simulink model "generic_Truck_And_Trailer"  (R2025a)
settings: Solver=VariableStepAuto  StartTime=0.0  StopTime=350  FixedStep=0.01  MaxStep=0.001  RelTol=1e-3  EnableMultiTasking=on
libraries: TruckMaker4SL x250, simulink x1
(part 7 of 11)

== matlab function generic_Truck_And_Trailer/TruckMaker/Subsystem1/ONE_TRACK_MODEL_TRACTOR_UKF/UKF_ONE_TRACK_TruckAndTrailer ==
  data: z input; u input; xhat output; Q input; R input; Ts input; P output; dxdt output; innovation output; K_out output; S_out output; z_pred_out output; data input; truck_Ff output; truck_Fr output; trailer_v_hitch output; trailer_v_axle output; trailer_F_hitch output; trailer_F_tire output; truck_v_hitch output
function [xhat, P, dxdt, innovation, K_out, S_out, z_pred_out,truck_Ff,truck_Fr, trailer_v_hitch,trailer_v_axle,trailer_F_hitch,trailer_F_tire,truck_v_hitch] = UKF_TruckTrailer(z,u,Q,R,Ts,data)

persistent x Pk dxdt_old t
%% =========================
%% INIT
%% =========================
if isempty(x)
    x = [15;0.1;0.1;14;14;0;0;5]; % [vx vy wz Cf Cr psi wz_tr Cr_tr]
end
if isempty(Pk)
    Pk = diag([0.1 0.1 0.1 5 5 0.03 0.1 5]);
end
if isempty(dxdt_old)
    dxdt_old = zeros(8,1);
end
if isempty(t)
    t = 0;
end
t = data;
if t < 30
    xhat=x; P=Pk; dxdt=dxdt_old;
    
    innovation=zeros(length(z),1);
    K_out=zeros(length(x), length(z));
    S_out=eye(length(z));
    z_pred_out=zeros(length(z),1);
    
    trailer_v_axle   = zeros(3,1);
    trailer_v_hitch = zeros(3,1);
    truck_Ff = zeros(2,1);
    truck_Fr = zeros(2,1);
    truck_v_hitch=zeros(3,1);
    
    trailer_F_hitch = zeros(2,1);
    trailer_F_tire = zeros(2,1);
    
    return
end

%% =========================
%% CONSTANTS
%% =========================
g = 9.82;
% Truck
m = 6800; 
Jz = 12994.917; 
Rwheel = 0.50;
w_track = 2.1; 
% Trailer
m_tr = 31960;
Jz_tr = 145971.764;
% Geometry & koordinat punkter på Truck
p_cog = [3.473;0;0.925];
p_fax = [4.520;0;0.49];
p_rax = [0.950;0;0.49];
p_imu = [3.600;0;1.000];
hitch = [1.9;0;1.21];
Rcog = p_imu - p_cog;
hHitch= hitch(3);
lf = abs(p_fax(1)-p_cog(1)); 
lr = abs(p_cog(1)-p_rax(1)); 
L = lf + lr;
h = p_cog(3);
Rfax = p_fax - p_cog; Rfax(3)=-p_cog(3);
Rrax = p_rax - p_cog; Rrax(3)=-p_cog(3);
Rhitch = hitch - p_cog;
lhitch = Rhitch(1);
% Geometry Trailer
p_cog_tr = [-6.195;0;1.95];
p_rFax_tr = [-7.75;0;0.49];
p_rMax_tr = [-9.0;0;0.49];
p_rRax_tr = [-10.25;0;0.49];
hitch_tr = [-1.25;0;1.25];

% Avstånd från hitch till trailer-punkter
lf_h_tr = abs(hitch_tr(1)-p_cog_tr(1));
lr_f_tr = abs(p_cog_tr(1)-p_rFax_tr(1));
lr_m_tr = abs(p_cog_tr(1)-p_rMax_tr(1));
lr_r_tr = abs(p_cog_tr(1)-p_rRax_tr(1));
L_tr = lf_h_tr + lr_m_tr; % Hävarm till mittaxel

% Vektorer från trailer-CoG till axlar (för cross-product)
Frax_tr = p_rFax_tr - p_cog_tr; Frax_tr(3) = -p_cog_tr(3);
Mrax_tr = p_rMax_tr - p_cog_tr; Mrax_tr(3) = -p_cog_tr(3);
Rlrax_tr = p_rRax_tr - p_cog_tr; Rlrax_tr(3) =-p_cog_tr(3);
Rhitch_tr = hitch_tr - p_cog_tr; Rhitch_tr(3) = -abs(hitch_tr(3)-p_cog_tr(3));

h_cog_tr = p_cog_tr(3);

% Statisk load transfer parametrar (beräknas en gång)
l_1 = -lr_f_tr; l_2 = -lr_m_tr; l_3 = -lr_r_tr;
l_h = lf_h_tr;
mg_tr = m_tr * g;
denom = l_1 + l_2 + l_3 - 3*l_h;

%% =========================
%% INPUTS
%% =========================
delta = u(1); 
T_rl  = u(2);   
T_rr  = u(3);
Fxh   = u(4); 
Fx_f_brake  = -abs(u(6)) / Rwheel; 
Fx_r_brake  = -abs(u(7)) / Rwheel;
Fx_vehicle  = (T_rl+T_rr)/Rwheel + Fx_r_brake +Fx_f_brake;

%% =========================
%% UKF PARAMS
%% =========================
n = length(x);
nSPx = 2*n+1;
W0 = 1 - n/3;
Wi = (1 - W0)/(2*n);
gamma = sqrt(n/(1 - W0));

%% =========================
%% SIGMA POINTS (PRIOR)
%% =========================
Pk = (Pk+Pk')/2 + 1e-9*eye(n);
Sx = chol(Pk,'lower');
X_pre = zeros(n,nSPx);
X_pre(:,1) = x;
for i=1:n
    X_pre(:,i+1)   = x + gamma*Sx(:,i);
    X_pre(:,i+1+n) = x - gamma*Sx(:,i);
end

%% =========================
%% PREDICTION
%% =========================
X_pred = zeros(n,nSPx);
dxdt_model = zeros(n,1);
truck_Ff = zeros(2,1);
truck_Fr = zeros(2,1);
truck_v_hitch = zeros(3,1);
    
trailer_v_axle = zeros(3,1);
trailer_v_hitch = zeros(3,1);
trailer_F_hitch = zeros(2,1);
trailer_F_tire = zeros(2,1);

for k=1:nSPx
    Xk = X_pre(:,k);
    vx=Xk(1); vy=Xk(2); wz=Xk(3); Cf=Xk(4); Cr=Xk(5);
    psi=Xk(6); wz_tr=Xk(7); Cr_tr=Xk(8);
    
    v_cog=[vx;vy;0];
    omega=[0;0;wz];
    
    %% ===== TRAILER =====
    v_hitch_truck = v_cog + cross(omega,Rhitch);
    
    Rot_tr=[cos(psi) -sin(psi) 0;
            sin(psi) cos(psi)  0; 
              0         0      1];
   
    v_hitch_trailer = Rot_tr' * v_hitch_truck;
    
    % *** STATISK LOAD TRANSFER (Axels metod) ***
    Fz_hitch = (mg_tr * (l_1 + l_2 + l_3)) / denom;
    Fz_tr_each = -(l_h * mg_tr) / denom;
    
    % Begränsa till fysiska värden
    Fz_hitch = max(100, min(Fz_hitch, m_tr*g));
    Fz_tr_each = max(100, min(Fz_tr_each, m_tr*g));

    % Hastigheter och slip för traileraxlar (relativt trailer CoG)
    omega_tr = [0;0;wz_tr];
    v_cog_tr = v_hitch_trailer - cross(omega_tr, Rhitch_tr);
    
    v_tr_f = v_cog_tr + cross(omega_tr, Frax_tr);
    v_tr_m = v_cog_tr + cross(omega_tr, Mrax_tr);
    v_tr_r = v_cog_tr + cross(omega_tr, Rlrax_tr);  
    
    alpha_tr_f = atan2(v_tr_f(2), max(abs(v_tr_f(1)), 0.1));
    alpha_tr_m = atan2(v_tr_m(2), max(abs(v_tr_m(1)), 0.1));
    alpha_tr_r = atan2(v_tr_r(2), max(abs(v_tr_r(1)), 0.1));
    
    Fy_f_tr = -Cr_tr * alpha_tr_f * Fz_tr_each;
    Fy_m_tr = -Cr_tr * alpha_tr_m * Fz_tr_each;
    Fy_r_tr = -Cr_tr * alpha_tr_r * Fz_tr_each;
    
    % Hitch-kraft (momentjämvikt)
    Fyh_mod = (Fy_f_tr*lr_f_tr + Fy_m_tr*lr_m_tr + Fy_r_tr*lr_r_tr) / (L_tr);
     
    if k==1
        trailer_v_hitch = v_hitch_trailer;
        trailer_v_axle = v_tr_m;
        truck_v_hitch = v_hitch_truck;
        trailer_F_hitch = [Fyh_mod; Fz_hitch];
        trailer_F_tire = [Fy_m_tr; Fz_tr_each];
    end

    %% ===== TRUCK =====
    % Transformera hitch-krafter till Truckens system
    F_hitch_body = Rot_tr * [Fxh; Fyh_mod; 0];
    
    Rotf=[cos(delta) -sin(delta)  0; 
          sin(delta)  cos(delta)  0;
              0           0       1];
    vf = Rotf'*(v_cog + cross(omega,Rfax));
    vr = v_cog + cross(omega,Rrax);
    
    alpha_f = atan2(vf(2),max(abs(vf(1)),0.1));
    alpha_r = atan2(vr(2),max(abs(vr(1)),0.1));
    
    % Vertikallast Truck
    ax_est = (Fx_vehicle - F_hitch_body(1))/m; 
    Ffz = (m*g*lr - m*ax_est*h + Fz_hitch*(hitch(1) - p_rax(1)) - F_hitch_body(1)*hHitch) / L;
    Frz = (m*g*lf + m*ax_est*h + Fz_hitch*(p_fax(1) - hitch(1)) + F_hitch_body(1)*hHitch) / L;
    
    Fy_f = -Cf * alpha_f * Ffz;
    Fy_r = -Cr * alpha_r * Frz;
    
    %% ===== DYNAMICS =====
    dvx = (Fx_vehicle - Fy_f*sin(delta) - F_hitch_body(1))/m + vy*wz;
    dvy = (Fy_f*cos(delta) + Fy_r - F_hitch_body(2))/m - vx*wz;
    dwz = (lf*Fy_f*cos(delta) - lr*Fy_r - lhitch*F_hitch_body(2))/Jz;
    
    dpsi = wz_tr - wz;  % Rätt tecken!
    
    % Moment kring trailer Cog
    dwz_tr = (lf_h_tr*Fyh_mod - lr_f_tr*Fy_f_tr - lr_m_tr*Fy_m_tr - lr_r_tr*Fy_r_tr)/Jz_tr;
    
    if k==1
        dxdt_model=[dvx;dvy;dwz;0;0;dpsi;dwz_tr;0];
        truck_Ff = [Fy_f;Ffz];
        truck_Fr = [Fy_r;Frz];
    end
    X_pred(:,k) = Xk + Ts*[dvx; dvy; dwz; 0; 0; dpsi; dwz_tr; 0];
end

%% ===== MEAN & COV
x_pred=zeros(n,1);
for k=1:nSPx
    w=(k==1)*W0+(k>1)*Wi;
    x_pred=x_pred+w*X_pred(:,k);
end
P_pred=zeros(n);
for k=1:nSPx
    w=(k==1)*W0+(k>1)*Wi;
    dx=X_pred(:,k)-x_pred;
    P_pred=P_pred+w*(dx*dx');
end
P_pred=P_pred+Q*Ts;

%% =========================
%% MEASUREMENT UPDATE
%% =========================
Sx=chol((P_pred+P_pred')/2 + 1e-9*eye(n),'lower');
X_post=zeros(n,nSPx);
X_post(:,1)=x_pred;
for i=1:n
    X_post(:,i+1)  =x_pred + gamma*Sx(:,i);
    X_post(:,i+1+n)=x_pred - gamma*Sx(:,i);
end

Z=zeros(10,nSPx);
for k=1:nSPx
    Xk=X_post(:,k);
    vx=Xk(1); vy=Xk(2); wz=Xk(3); Cf=Xk(4); Cr=Xk(5);
    psi=Xk(6); wz_tr=Xk(7); Cr_tr=Xk(8); 

    v_cog=[vx;vy;0];
    omega=[0;0;wz];
    
    % *** SAMMA STATISKA LOAD TRANSFER som i prediction ***
    Fz_hitch_meas = (mg_tr * (l_1 + l_2 + l_3)) / denom;
    Fz_tr_each_meas = -(l_h * mg_tr) / denom;
    
    Fz_hitch_meas = max(100, min(Fz_hitch_meas, m_tr*g));
    Fz_tr_each_meas = max(100, min(Fz_tr_each_meas, m_tr*g));
    
    % Upprepa kraftberäkning för z_pred
    Rot_tr=[cos(psi) -sin(psi) 0;
            sin(psi)  cos(psi) 0;
                0       0      1];

    v_hitch_tr = Rot_tr' * ([vx;vy;0] + cross([0;0;wz],Rhitch));
    
    % Samma logik som i prediction
    v_cog_tr_meas = v_hitch_tr - cross([0;0;wz_tr], Rhitch_tr);
    v_tr_m_meas = v_cog_tr_meas + cross([0;0;wz_tr], Mrax_tr);
    alpha_tr_m = atan2(v_tr_m_meas(2), max(abs(v_tr_m_meas(1)), 0.1));
    Fy_m_tr_meas = -Cr_tr * alpha_tr_m * Fz_tr_each_meas;
   
    % Beräkna Fy_f_tr och Fy_r_tr för hitch-kraften
    v_tr_f_meas = v_cog_tr_meas + cross([0;0;wz_tr], Frax_tr);
    v_tr_r_meas = v_cog_tr_meas + cross([0;0;wz_tr], Rlrax_tr);
    alpha_tr_f_meas = atan2(v_tr_f_meas(2), max(abs(v_tr_f_meas(1)), 0.1));
    alpha_tr_r_meas = atan2(v_tr_r_meas(2), max(abs(v_tr_r_meas(1)), 0.1));
    Fy_f_tr_meas = -Cr_tr * alpha_tr_f_meas * Fz_tr_each_meas;
    Fy_r_tr_meas = -Cr_tr * alpha_tr_r_meas * Fz_tr_each_meas;
    
    % Hitch-kraft (momentjämvikt)
    Fyh_mod_meas = (Fy_f_tr_meas*lr_f_tr + Fy_m_tr_meas*lr_m_tr + Fy_r_tr_meas*lr_r_tr) / L_tr;

    
    F_hitch_body = Rot_tr * [Fxh; Fyh_mod_meas; 0];
    
    % Vertikallast Truck för measurement
    ax_est_meas = (Fx_vehicle - F_hitch_body(1))/m; 
    Ffz_meas = (m*g*lr - m*ax_est_meas*h + Fz_hitch_meas*(hitch(1) - p_rax(1)) - F_hitch_body(1)*hHitch) / L;
    Frz_meas = (m*g*lf + m*ax_est_meas*h + Fz_hitch_meas*(p_fax(1) - hitch(1)) + F_hitch_body(1)*hHitch) / L;

    Rotf=[cos(delta) -sin(delta)  0; 
          sin(delta)  cos(delta)  0;
              0           0       1];
    vf = Rotf'*(v_cog + cross(omega,Rfax));
    vr = v_cog + cross(omega,Rrax);
    
    alpha_f = atan2(vf(2),max(abs(vf(1)),0.1));
    alpha_r = atan2(vr(2),max(abs(vr(1)),0.1));
    
    %alpha_f = atan2(vy + lf*wz, max(abs(vx),0.1)) - delta;
    %alpha_r = atan2(vy - lr*wz, max(abs(vx),0.1));
    Fy_f_meas = -Cf * alpha_f * Ffz_meas;
    Fy_r_meas = -Cr * alpha_r * Frz_meas;
    
    a_spec_x = (Fx_vehicle - Fy_f_meas*sin(delta) - F_hitch_body(1))/m;
    a_spec_y = (Fy_f_meas*cos(delta) + Fy_r_meas - F_hitch_body(2))/m;
    dwz_m = (lf*Fy_f_meas*cos(delta) - lr*Fy_r_meas - lhitch*F_hitch_body(2))/Jz;
    
    a_imu = [a_spec_x; a_spec_y; 0] + cross([0;0;wz],cross([0;0;wz],Rcog)) + cross([0;0;dwz_m],Rcog);
    v_imu = [vx;vy;0] + cross([0;0;wz],Rcog);
    
    Z(:,k)=[a_imu(1:2); v_imu(1); v_imu(2); wz; ...
            (vx - wz*w_track/2)/Rwheel; (vx + wz*w_track/2)/Rwheel; ...
            (v_tr_m_meas(1) - wz_tr*w_track/2)/Rwheel; (v_tr_m_meas(1) + wz_tr*w_track/2)/Rwheel; Fyh_mod_meas];
end

z_pred=zeros(10,1);
for k=1:nSPx
    w=(k==1)*W0+(k>1)*Wi;
    z_pred=z_pred+w*Z(:,k);
end

valid_idx = ~isnan(z);
z_used = z(valid_idx);
z_pred_used = z_pred(valid_idx);
R_used = R(valid_idx,valid_idx);

S_cov=zeros(length(z_used));
Pxz=zeros(n,length(z_used));
for k=1:nSPx
    w=(k==1)*W0+(k>1)*Wi;
    dz=Z(valid_idx,k)-z_pred_used;
    dx=X_post(:,k)-x_pred;
    S_cov=S_cov+w*(dz*dz');
    Pxz=Pxz+w*(dx*dz');
end
S_cov=S_cov+R_used;
K=Pxz/S_cov;

x=x_pred + K*(z_used - z_pred_used);
Pk=P_pred - K*S_cov*K';
Pk=(Pk+Pk')/2 + 1e-9*eye(n);

%% OUTPUT
xhat=x; P=Pk; dxdt=dxdt_model;
innovation=zeros(length(z),1); innovation(valid_idx)=z_used - z_pred_used;
K_out=zeros(n,length(z)); K_out(:,valid_idx)=K;
S_out=zeros(length(z)); S_out(valid_idx,valid_idx)=S_cov;
z_pred_out=z_pred;

end

== matlab function generic_Truck_And_Trailer/TruckMaker/Subsystem1/EKF_ONE_TRACK ==
  data: z input; u input; xhat output; Q input; R input; Ts input; P output
function [xhat, P] = EKF_Bicycle_Full_NoBias(z, u, Q, R, Ts)
% EKF for One-Track / Bicycle Model (No IMU Bias)
% States: x = [vx; vy; r; Cf; Cr]
% Measurements: z = [ax; ay; vx; vy; r; wL; wR]

%% ---------------- Persistent safe initialization ----------------
persistent x Pk initialized

% Säker initialisering
if isempty(x)
    x = [15; 0; 0.05; 2e4; 2e4];  % vx, vy, r, Cf, Cr
end

if isempty(Pk)
    Pk = diag([1 1 0.05 4e4 4e4].^2); % 5x5
end

if isempty(initialized)
    initialized = true;
end


%% ---------------- Vehicle parameters ----------------

m  = 6800;        %  mass
g  = 9.82;        % gravity contanst   
Jz = 12994.917;   % yaw interia
Rw = 0.49;          % wheel radius
width = 2.49;       % track width

p_cog  = [3.473; 0; 0.925];
p_fax  = [4.520; 0; 0.490];

p_rax  = [0.950; 0; 0.490];
p_imu  = [3.600; 0; 1.000];

lf = abs(p_fax(1)-p_cog(1));   % front CoG distance
lr = abs(p_cog(1)-p_rax(1));   % rear CoG distance
L  = lf + lr;
h  = p_cog(3);

Rfax = p_fax - p_imu; Rfax(3) = -p_imu(3);
Rrax = p_rax - p_imu; Rrax(3) = -p_imu(3);
Rcog = p_cog - p_imu;

%% ---------------- Inputs ----------------
delta = u(1);                             % Average steering Angle (FL +FR)/2
T_rl  = u(2);                             % torque RL  
T_rr  = u(3);                             %torque RR
Rwheel = 0.49;                            % wheel radius
Fx_vehicle = (T_rl + T_rr)/Rwheel;        % longitudinal force

%% ---------------- States ----------------
vx = x(1); vy = x(2); r = x(3); Cf = x(4); Cr= x(5);

Rotf = [ cos(delta)     -sin(delta)     0;
         sin(delta)      cos(delta)     0;
             0              0           1];

v_cog = [vx; vy; 0];
omega = [0;0;r];

% Contact patch velocities
vf = Rotf.' * (v_cog + cross(omega,Rfax));
vr = v_cog + cross(omega,Rrax);

alpha_f = atan2(vf(2), max(abs(vf(1)),0.1));
alpha_r = atan2(vr(2), max(abs(vr(1)),0.1));

% Longitudinal accel estimate to compute the vertikel forces
dvx_temp = Fx_vehicle/m + vy*r;

% Normal forces
Ffz = m*g*lr/L - m*dvx_temp*h/L;
Frz = m*g*lf/L + m*dvx_temp*h/L;

% Tire forces
Fy_f = Cf * alpha_f * Ffz;
Fy_r = Cr * alpha_r * Frz;

% Full dynamics 
dvx = (Fx_vehicle - Fy_f*sin(delta))/m + vy*r;
dvy = (Fy_f*cos(delta) + Fy_r)/m - vx*r;
dr  = (lf*Fy_f*cos(delta) - lr*Fy_r)/Jz;

% State propagation
xdot = [dvx; dvy; dr; 0; 0];
x_pred = x + Ts*xdot;

%% ---------------- Jacobian F ----------------
F= zeros(5,5);
F(1,:) = [                                1 - (Cf*Ts*sin(delta)*(vy + lf*r))/(m*vx^2),              Ts*(r + (Cf*sin(delta))/(m*vx)),                   Ts*(vy + (Cf*lf*sin(delta))/(m*vx)),    -(Ts*sin(delta)*(delta - (vy + lf*r)/vx))/m,                            0];
F(2,:) = [  -Ts*(r - ((Cr*(vy - lr*r))/vx^2 + (Cf*cos(delta)*(vy + lf*r))/vx^2)/m),      1 - (Ts*(Cr/vx + (Cf*cos(delta))/vx))/m,    -Ts*(vx - ((Cr*lr)/vx - (Cf*lf*cos(delta))/vx)/m),     (Ts*cos(delta)*(delta - (vy + lf*r)/vx))/m,    -(Ts*(vy - lr*r))/(m*vx)];
F(3,:) = [-(Ts*((Cr*lr*(vy - lr*r))/vx^2 - (Cf*lf*cos(delta)*(vy + lf*r))/vx^2))/Jz, (Ts*((Cr*lr)/vx - (Cf*lf*cos(delta))/vx))/Jz, 1 - (Ts*((Cf*cos(delta)*lf^2)/vx + (Cr*lr^2)/vx))/Jz, (Ts*lf*cos(delta)*(delta - (vy + lf*r)/vx))/Jz, (Ts*lr*(vy - lr*r))/(Jz*vx)];
F(4,:) = [                                                                            0,                                              0,                                                      0,                                                 1,                            0];
F(5,:) = [                                                                            0,                                              0,                                                      0,                                                 0,                            1];


%% ---------------- Covariance prediction ----------------
P_pred = F*Pk*F' + Q;

%% ---------------- Measurement model ----------------
ax_hat = dvx -  vy*r;                % longitudinal accel
ay_hat = dvy + vx*r;                % lateral accel
%vx_hat = vx;
%vy_hat = vy;
%r_hat  = r;
%wL_hat = (vx - width/2 * r)/Rw;
%wR_hat = (vx + width/2 * r)/Rw;

a_cog = [ax_hat; ay_hat; 0];
alpha_vec = [0;0;dr];

% Transform to IMU
a_imu = a_cog - cross(omega, cross(omega,Rcog))- cross(alpha_vec,Rcog);
v_imu = v_cog + cross(omega,Rcog);

z_hat = [a_imu(1:2);
         v_imu(1:2);
         alpha_vec(3);
         omega(3)];

%z_hat = [ax_hat; ay_hat; vx_hat; vy_hat; dr_hat r_hat; wL_hat; wR_hat];

%% ---------------- Measurement Jacobian H ----------------
H = zeros(size(z_hat,1),size(x,1));

%H = zeros(7,5);
H(1,:) = [                               1 - (Cf*Ts*sin(delta)*(vy + lf*r))/(m*vx^2),         Ts*(r + (Cf*sin(delta))/(m*vx)) - r,                      Ts*(vy + (Cf*lf*sin(delta))/(m*vx)) - vy, -(Ts*sin(delta)*(delta - (vy + lf*r)/vx))/m,                            0];
H(2,:) = [-Ts*(r - ((Cr*(vy - lr*r))/vx^2 + (Cf*cos(delta)*(vy + lf*r))/vx^2)/m), 1 - (Ts*(Cr/vx + (Cf*cos(delta))/vx))/m, vx - Ts*(vx - ((Cr*lr)/vx - (Cf*lf*cos(delta))/vx)/m),  (Ts*cos(delta)*(delta - (vy + lf*r)/vx))/m, -(Ts*(vy - lr*r))/(m*vx)];
H(3,:) = [                                                                             1,                                               0,                                                                 0,                                               0,            0];
H(4,:) = [                                                                             0,                                               1,                                                                 0,                                               0,            0];
H(5,:) = [                                                                             0,                                               0,                                                                 0,                                               0,            0];
H(6,:) = [                                                                             0,                                               0,                                                                 1,                                               0,            0];
%H(7,:) = [                                                                             1/Rw,                                            0,                                                     -width/(2*Rw),                                               0,            0];
%H(8,:) = [                                                                             1/Rw,                                            0,                                                      width/(2*Rw),                                               0,            0];

%% ---------------- EKF update ----------------
S = H*P_pred*H' + R;
K = P_pred*H'/(S + 1e-9*eye(size(S)));

x = x_pred + K*(z - z_hat);
Pk = P_pred - K*S*K';

%% ---------------- Output ----------------
xhat = x;
P = Pk;

end

== matlab function generic_Truck_And_Trailer/TruckMaker/UKF_Articulated_Vehicles ==
  data: z input; u input; xhat output; Q input; R input; Ts input; P output
function [xhat,P] = UKF_TruckTrailer_Robust(z,u,Q,R,Ts)

persistent x Pk

%% INITIALIZATION

if isempty(x)

    % [vx vy r theta Cf Cr Ct]

    x = [15;0.1;0.01;0;5;5;5];

end

if isempty(Pk)

    Pk = diag([1 1 0.1 0.01 5 5 5]);

end


%% PARAMETERS (fill from TruckMaker later)

m  = PARAM.m;
Jz = PARAM.Jz;

mt = PARAM.mt;

lf = PARAM.lf;
lr = PARAM.lr;

lh = PARAM.lh;     % hitch distance
lt = PARAM.lt;     % trailer axle distance

g = 9.82;


%% INPUTS

delta = u(1);
Fx    = u(2);

ay_meas = z(2);


%% EXCITATION CHECK

excitation = abs(ay_meas) > 0.3 && abs(delta) > 0.5*pi/180;


%% UKF PARAMETERS

n = length(x);

W0 = 1 - n/3;
Wi = (1-W0)/(2*n);
gamma = sqrt(n/(1-W0));

Pk = (Pk+Pk')/2 + 1e-9*eye(n);

S = chol(Pk,'lower');


%% SIGMA POINTS

X = zeros(n,2*n+1);
X(:,1) = x;

for i=1:n

    X(:,i+1)   = x + gamma*S(:,i);
    X(:,i+1+n) = x - gamma*S(:,i);

end


%% PROPAGATION

X_pred = zeros(n,2*n+1);

for k=1:2*n+1

vx = X(1,k);
vy = X(2,k);
r  = X(3,k);
theta = X(4,k);

Cf = X(5,k);
Cr = X(6,k);
Ct = X(7,k);


%% SLIP ANGLES

alpha_f = delta - atan2(vy + lf*r , max(vx,0.5));

alpha_r = -atan2(vy - lr*r , max(vx,0.5));

alpha_t = -atan2(vy - (lr+lt)*r + lh*r , max(vx,0.5));


%% NORMAL FORCES

Ffz = PARAM.Ffz;
Frz = PARAM.Frz;

Ftz = PARAM.Ftz;


%% LATERAL FORCES

Fy_f = Cf * alpha_f * Ffz;

Fy_r = Cr * alpha_r * Frz;

Fy_t = Ct * alpha_t * Ftz;


%% VEHICLE DYNAMICS

dvx = Fx/m + vy*r;

dvy = (Fy_f*cos(delta) + Fy_r + Fy_t)/(m+mt) - vx*r;

dr  = (-lf*Fy_f*cos(delta) + lr*Fy_r - lh*Fy_t)/Jz;


%% ARTICULATION

dtheta = r - (vy - (lr+lt)*r)/lh;


%% PROPAGATION

X_pred(:,k) = [

vx + Ts*dvx
vy + Ts*dvy
r  + Ts*dr
theta + Ts*dtheta
Cf
Cr
Ct

];

end


%% MEAN

x_pred = W0*X_pred(:,1);

for k=2:2*n+1

x_pred = x_pred + Wi*X_pred(:,k);

end


%% COVARIANCE

P_pred = Q;

for k=1:2*n+1

w = (k==1)*W0 + (k>1)*Wi;

dx = X_pred(:,k)-x_pred;

P_pred = P_pred + w*(dx*dx');

end


%% MEASUREMENT MODEL

Z = zeros(length(z),2*n+1);

for k=1:2*n+1

vx = X_pred(1,k);
vy = X_pred(2,k);
r  = X_pred(3,k);

ax = Fx/m + vy*r;

ay = -vx*r;

Z(:,k) = [

ax
ay
vx
vy
r

];

end


%% MEASUREMENT MEAN

z_pred = W0*Z(:,1);

for k=2:2*n+1

z_pred = z_pred + Wi*Z(:,k);

end


%% MEASUREMENT COV

S_cov = R;

for k=1:2*n+1

w = (k==1)*W0 + (k>1)*Wi;

dz = Z(:,k)-z_pred;

S_cov = S_cov + w*(dz*dz');

end


%% CROSS COV

Pxz = zeros(n,length(z));

for k=1:2*n+1

w = (k==1)*W0 + (k>1)*Wi;

dx = X_pred(:,k)-x_pred;

dz = Z(:,k)-z_pred;

Pxz = Pxz + w*(dx*dz');

end


%% UPDATE

K = Pxz / S_cov;

x = x_pred + K*(z - z_pred);

Pk = P_pred - K*S_cov*K';


%% ROBUST CONSTRAINTS

x(5) = min(max(x(5),0.01),20);   % Cf

x(6) = min(max(x(6),0.01),20);   % Cr

x(7) = min(max(x(7),0.01),20);   % Ct


%% EXCITATION FREEZE

if ~excitation

x(5:7) = x_pred(5:7);

end


%% ARTICULATION LIMIT

if abs(x(4)) > 20*pi/180

x(7) = x_pred(7);

end


xhat = x;

P = Pk;

end

== matlab function generic_Truck_And_Trailer/TruckMaker/MATLAB Function ==
  data: u input; y output
function y = fcn(u)

y = u;

== matlab function generic_Truck_And_Trailer/TruckMaker/Subsystem1/Subsystem/Ackerman Angle/MATLAB Function ==
  data: delta_l input; delta output; delta_r input
function delta = ackerman_angle(delta_l, delta_r)

delta = acot((cot(delta_l) + cot(delta_r))/2);

end

== matlab function generic_Truck_And_Trailer/TruckMaker/Subsystem1/Subsystem_Noisey Measurements/MATLAB Function ==
  data: gyro_true input; gyro_meas output
function gyro_meas = imu_gyro_noise(gyro_true)

Fs = 1000;   % sample rate

[meas, ~] = GyroNoise(gyro_true', Fs);

gyro_meas = meas';

end

== matlab function generic_Truck_And_Trailer/TruckMaker/Subsystem1/Subsystem_Noisey Measurements/MATLAB Function1 ==
  data: acc_true input; acc_meas output
function acc_meas = AccelNoiseBlock(acc_true)

Fs = 1000;

truth = acc_true;      % 1×3

[meas,~] = AccelNoise(truth,Fs);

acc_meas = meas;       % 3×1

end

== matlab function generic_Truck_And_Trailer/TruckMaker/Subsystem1/Subsystem_Noisey Measurements/MATLAB Function2 ==
  data: truth input; vel_meas output
function vel_meas = imu_vel_noise(truth)
    

sigma = 0.05; % m/s^2 (tune later)

vel_meas = truth + sigma * randn(size(truth));


end

== matlab function generic_Truck_And_Trailer/TruckMaker/Subsystem1/ONE_TRACK_MODEL_TRACTOR_UKF/Working Model with 5 measurements  ==
  data: z input; u input; xhat output; Q input; R input; Ts input; P output; dxdt output; innovation output; K_out output; S_out output; z_pred_out output
function [xhat, P, dxdt, innovation, K_out, S_out, z_pred_out] = UKF_OneTrack_IMU(z, u, Q, R, Ts)

% z = [ax; ay; vx; vy; wz]

%% =========================
%% PERSISTENT VARIABLES
%% =========================
persistent x Pk dxdt_old t

if isempty(x)
    x = [15;0.1;0.1;7.5;7.5];   % [vx vy wz Cf Cr]
end
if isempty(Pk)
    Pk = diag([0.1 0.1 0.1 2 2]);
end
if isempty(dxdt_old)
    dxdt_old = zeros(5,1);
end
if isempty(t)
    t = 0;
end

%% =========================
%% TIME UPDATE
%% =========================
t = t + 0.001;

start_time = 30;
if t < start_time
    xhat = x;
    P = Pk;
    dxdt = dxdt_old;

    innovation = zeros(length(z),1);
    K_out = zeros(length(x), length(z));
    S_out = eye(length(z));
    z_pred_out = zeros(length(z),1);
    return
end

%% =========================
%% VEHICLE PARAMETERS
%% =========================
m  = 6800;
g  = 9.82;
Jz = 12994.917;

p_cog = [3.473;0;0.925];
p_fax = [4.520;0;0.490];
p_rax = [0.950;0;0.490];
p_imu = [3.600;0;1.000];

lf = abs(p_fax(1)-p_cog(1));
lr = abs(p_cog(1)-p_rax(1));
L  = lf + lr;
h  = p_cog(3);

Rfax = p_fax - p_cog; Rfax(3) = -p_cog(3);
Rrax = p_rax - p_cog; Rrax(3) = -p_cog(3);
Rcog = p_imu - p_cog;

%% =========================
%% INPUTS
%% =========================
delta = u(1);
T_rl  = u(2);
T_rr  = u(3);
Rwheel = 0.505;

Fx_vehicle = (T_rl + T_rr)/(Rwheel);

%% =========================
%% UKF PARAMETERS
%% =========================
n = length(x);
W0 = 1 - n/3;
Wi = (1 - W0)/(2*n);
gamma = sqrt(n/(1-W0));

Pk = (Pk+Pk')/2 + 1e-9*eye(n);
S = chol(Pk,'lower');

%% =========================
%% SIGMA POINTS
%% =========================
X = zeros(n,2*n+1);
X(:,1) = x;

for i=1:n
    X(:,i+1)   = x + gamma*S(:,i);
    X(:,i+1+n) = x - gamma*S(:,i);
end

%% =========================
%% PREDICTION
%% =========================
X_pred = zeros(n,2*n+1);
dxdt_model = zeros(5,1);

for k=1:2*n+1

    vx = X(1,k);
    vy = X(2,k);
    wz = X(3,k);
    Cf = X(4,k);
    Cr = X(5,k);

    v_cog = [vx;vy;0];
    omega = [0;0;wz];

    Rotf = [cos(delta) -sin(delta) 0;
            sin(delta)  cos(delta) 0;
            0 0 1];

    vf = Rotf.'*(v_cog + cross(omega,Rfax));
    vr = v_cog + cross(omega,Rrax);

    alpha_f = atan2(vf(2), max(abs(vf(1)),0.1));
    alpha_r = atan2(vr(2), max(abs(vr(1)),0.1));

    ax_est = Fx_vehicle/m + vy*wz;

    Ffz = m*g*lr/L - m*ax_est*h/L;
    Frz = m*g*lf/L + m*ax_est*h/L;

    Fy_f = -Cf * alpha_f * Ffz;
    Fy_r = -Cr * alpha_r * Frz;

    dvx = (Fx_vehicle - Fy_f*sin(delta))/m + vy*wz;
    dvy = (Fy_f*cos(delta) + Fy_r)/m - vx*wz;
    dwz = (lf*Fy_f*cos(delta) - lr*Fy_r)/Jz;

    if k==1
        dxdt_model = [dvx; dvy; dwz; 0; 0];
    end

    X_pred(:,k) = [
        vx + Ts*dvx
        vy + Ts*dvy
        wz + Ts*dwz
        Cf
        Cr
    ];
end

%% =========================
%% MEAN + COV
%% =========================
x_pred = W0*X_pred(:,1);
for k=2:2*n+1
    x_pred = x_pred + Wi*X_pred(:,k);
end

P_pred = zeros(n);
for k=1:2*n+1
    w = (k==1)*W0 + (k>1)*Wi;
    dx = X_pred(:,k)-x_pred;
    P_pred = P_pred + w*(dx*dx');
end
P_pred = P_pred + Q*Ts;

%% =========================
%% MEASUREMENT MODEL
%% =========================
Z = zeros(length(z),2*n+1);

for k=1:2*n+1

    vx = X_pred(1,k);
    vy = X_pred(2,k);
    wz = X_pred(3,k);
    Cf = X_pred(4,k);
    Cr = X_pred(5,k);

    v_cog = [vx;vy;0];
    omega = [0;0;wz];

    Rotf = [cos(delta) -sin(delta) 0;
            sin(delta)  cos(delta) 0;
            0 0 1];

    vf = Rotf.'*(v_cog + cross(omega,Rfax));
    vr = v_cog + cross(omega,Rrax);

    alpha_f = atan2(vf(2), max(abs(vf(1)),0.1));
    alpha_r = atan2(vr(2), max(abs(vr(1)),0.1));

    ax_est = Fx_vehicle/m + vy*wz;

    Ffz = m*g*lr/L - m*ax_est*h/L;
    Frz = m*g*lf/L + m*ax_est*h/L;

    Fy_f = -Cf * alpha_f * Ffz;
    Fy_r = -Cr * alpha_r * Frz;

    dvx = (Fx_vehicle - Fy_f*sin(delta))/m;
    dvy = (Fy_f*cos(delta) + Fy_r)/m;
    dwz = (lf*Fy_f*cos(delta) - lr*Fy_r)/Jz;

    a_cog = [dvx; dvy; 0];
    alpha_vec = [0;0;dwz];

    a_imu = a_cog + cross(omega,cross(omega,Rcog)) + cross(alpha_vec,Rcog);
    v_imu = v_cog + cross(omega,Rcog);

    Z(:,k) = [a_imu(1:2); v_imu(1:2); wz];
end

%% =========================
%% HANDLE NaN MEASUREMENTS
%% =========================
valid_idx = ~isnan(z);

z_used      = z(valid_idx);
z_pred      = W0*Z(:,1);
for k=2:2*n+1
    z_pred = z_pred + Wi*Z(:,k);
end

z_pred_used = z_pred(valid_idx);
Z_used      = Z(valid_idx,:);
R_used      = R(valid_idx, valid_idx);

%% =========================
%% S
%% =========================
S_cov = zeros(length(z_used));
for k=1:2*n+1
    w = (k==1)*W0 + (k>1)*Wi;
    dz = Z_used(:,k)-z_pred_used;
    S_cov = S_cov + w*(dz*dz');
end
S_cov = S_cov + R_used;

%% =========================
%% Pxz
%% =========================
Pxz = zeros(n,length(z_used));
for k=1:2*n+1
    w = (k==1)*W0 + (k>1)*Wi;
    dx = X_pred(:,k)-x_pred;
    dz = Z_used(:,k)-z_pred_used;
    Pxz = Pxz + w*(dx*dz');
end

%% =========================
%% UPDATE
%% =========================
K = Pxz / S_cov;

x = x_pred + K*(z_used - z_pred_used);
Pk = P_pred - K*S_cov*K';
Pk = (Pk+Pk')/2 + 1e-9*eye(n);

%% =========================
%% OUTPUTS
%% =========================
dxdt_old = dxdt_model;

xhat = x;
P = Pk;
dxdt = dxdt_old;

innovation = zeros(length(z),1);
innovation(valid_idx) = z_used - z_pred_used;

K_out = zeros(n,length(z));
K_out(:,valid_idx) = K;

S_out = zeros(length(z));
S_out(valid_idx,valid_idx) = S_cov;

z_pred_out = z_pred;

end

== matlab function generic_Truck_And_Trailer/TruckMaker/Subsystem1/Subsystem_Noisey Measurements _NAN/MATLAB Function ==
  data: gyro_true input; gyro_meas output
function gyro_meas = imu_gyro_noise(gyro_true)

Fs = 1000;   % sample rate

[meas, ~] = GyroNoise(gyro_true', Fs);

gyro_meas = meas';

end

== matlab function generic_Truck_And_Trailer/TruckMaker/Subsystem1/Subsystem_Noisey Measurements _NAN/MATLAB Function1 ==
  data: acc_true input; acc_meas output
function acc_meas = AccelNoiseBlock(acc_true)

Fs = 1000;

truth = acc_true;      % 1×3

[meas,~] = AccelNoise(truth,Fs);

acc_meas = meas;       % 3×1

end

== matlab function generic_Truck_And_Trailer/TruckMaker/Subsystem1/Subsystem_Noisey Measurements _NAN/MATLAB Function2 ==
  data: truth input; vel_meas output
function vel_meas = imu_vel_noise(truth)
    

sigma = 0.05; % m/s^2 (tune later)

vel_meas = truth + sigma * randn(size(truth));


end

== matlab function generic_Truck_And_Trailer/TruckMaker/Subsystem1/Subsystem_Noisey Measurements _NAN/MATLAB Function3 ==
  data: truth input; vel_meas output
function vel_meas = imu_vel_noise(truth)
    

sigma = 0.05; % m/s^2 (tune later)

vel_meas = truth + sigma * randn(size(truth));


end

== matlab function generic_Truck_And_Trailer/TruckMaker/Subsystem1/ONE_TRACK_MODEL_TRACTOR_UKF/Working Model with 7 measurements ==
  data: z input; u input; xhat output; Q input; R input; Ts input; P output; dxdt output; innovation output; K_out output; S_out output; z_pred_out output; data input
function [xhat, P, dxdt, innovation, K_out, S_out, z_pred_out] = UKF_OneTrack_IMU(z, u, Q, R, Ts,data)

persistent x Pk dxdt_old t p_nom Pp

if isempty(x)
    x = [15;0.1;0.1;7.5;7.5];
end
if isempty(Pk)
    Pk = diag([0.1 0.1 0.1 5 5]);
end
if isempty(dxdt_old)
    dxdt_old = zeros(5,1);
end
if isempty(t)
    t = 0;
end
if isempty(p_nom)
    p_nom = [6800; 12994.917];
    Pp = diag([5000, 20000]).^2;
end

T_sim = 0.001;
t = t + T_sim;
t=data;

if t < 30
    xhat = x;
    P = Pk;
    dxdt = dxdt_old;
    innovation = zeros(length(z),1);
    K_out = zeros(length(x), length(z));
    S_out = eye(length(z));
    z_pred_out = zeros(length(z),1);
    return
end

IDX_VX  = 3; 
IDX_WRL = 6; 
IDX_WRR = 7;

g  = 9.82;

p_cog = [3.473;0;0.925];
p_fax = [4.520;0;0.490];
p_rax = [0.950;0;0.490];
p_imu = [3.600;0;1.000];

lf = abs(p_fax(1)-p_cog(1));
lr = abs(p_cog(1)-p_rax(1));
L  = lf + lr;
h  = p_cog(3);

Rfax = p_fax - p_cog; Rfax(3) = -p_cog(3);
Rrax = p_rax - p_cog; Rrax(3) = -p_cog(3);
Rcog = p_imu - p_cog;

delta = u(1);
T_rl  = u(2);
T_rr  = u(3);
Rwheel = 0.505;
Fx_vehicle = (T_rl + T_rr)/Rwheel;

n  = length(x);
np = length(p_nom);
nSPx = 2*n + 1;
nSPp = 2*np;
nSP  = nSPx + nSPp;

W0 = 1 - (n + np)/3;
Wi = (1 - W0)/(2*(n + np));
gamma = sqrt((n + np)/(1 - W0));

%% ===== STATE SIGMA =====
Pk = (Pk + Pk')/2 + 1e-9*eye(n);
Sx = chol(Pk,'lower');

X = zeros(n,nSPx);
X(:,1) = x;
for i=1:n
    X(:,i+1)   = x + gamma*Sx(:,i);
    X(:,i+1+n) = x - gamma*Sx(:,i);
end

%% ===== PARAM SIGMA =====
Pp = (Pp + Pp')/2 + 1e-9*eye(np);
Sp = chol(Pp,'lower');

SPp = zeros(np,nSPp);
for i=1:np
    SPp(:,i)    = p_nom + gamma*Sp(:,i);
    SPp(:,i+np) = p_nom - gamma*Sp(:,i);
end

%% ===== PREDICTION =====
X_prop = zeros(n,nSP);
dxdt_model = zeros(5,1);

for k=1:nSP
    if k <= nSPx
        Xk = X(:,k); 
        pk = p_nom;
    else
        Xk = x; 
        pk = SPp(:,k-nSPx);
    end

    vx=Xk(1); vy=Xk(2); wz=Xk(3); Cf=Xk(4); Cr=Xk(5);
    m=pk(1); Jz=pk(2);

    v_cog=[vx;vy;0]; omega=[0;0;wz];
    Rotf=[cos(delta) -sin(delta) 0; sin(delta) cos(delta) 0; 0 0 1];

    vf=Rotf.'*(v_cog+cross(omega,Rfax));
    vr=v_cog+cross(omega,Rrax);

    alpha_f=atan2(vf(2),max(abs(vf(1)),0.1));
    alpha_r=atan2(vr(2),max(abs(vr(1)),0.1));

    ax_est=Fx_vehicle/m+vy*wz;

    Ffz=m*g*lr/L - m*ax_est*h/L;
    Frz=m*g*lf/L + m*ax_est*h/L;

    Fy_f=-Cf*alpha_f*Ffz;
    Fy_r=-Cr*alpha_r*Frz;

    dvx=(Fx_vehicle - Fy_f*sin(delta))/m + vy*wz;
    dvy=(Fy_f*cos(delta)+Fy_r)/m - vx*wz;
    dwz=(lf*Fy_f*cos(delta) - lr*Fy_r)/Jz;

    if k==1
        dxdt_model=[dvx;dvy;dwz;0;0];
    end

    X_prop(:,k)=[vx+Ts*dvx; vy+Ts*dvy; wz+Ts*dwz; Cf; Cr];
end

%% ===== MEAN =====
x_pred=zeros(n,1);
for k=1:nSP
    w=(k==1)*W0 + (k>1)*Wi;
    x_pred=x_pred + w*X_prop(:,k);
end

%% ===== COV =====
P_pred=zeros(n);
for k=1:nSPx
    w=(k==1)*W0 + (k>1)*Wi;
    dx=X_prop(:,k)-x_pred;
    P_pred=P_pred + w*(dx*dx');
end
P_pred=P_pred + Q*Ts;

%% ===== NEW SIGMA POINTS =====
P_pred=(P_pred+P_pred')/2 + 1e-9*eye(n);
Sx=chol(P_pred,'lower');

SPx_new=zeros(n,nSPx);
SPx_new(:,1)=x_pred;

for i=1:n
    SPx_new(:,i+1)=x_pred+gamma*Sx(:,i);
    SPx_new(:,i+1+n)=x_pred-gamma*Sx(:,i);
end

%% ===== MEASUREMENT =====
Z=zeros(length(z),nSP);

for k=1:nSP
    if k<=nSPx
        Xk=SPx_new(:,k);
        pk=p_nom;
    else
        Xk=x_pred;
        pk=SPp(:,k-nSPx);
    end

    vx=Xk(1); vy=Xk(2); wz=Xk(3);
    Cf=Xk(4); Cr=Xk(5);

    m=pk(1); Jz=pk(2);

    v_cog=[vx;vy;0]; omega=[0;0;wz];
    Rotf=[cos(delta) -sin(delta) 0; sin(delta) cos(delta) 0; 0 0 1];

    vf=Rotf.'*(v_cog+cross(omega,Rfax));
    vr=v_cog+cross(omega,Rrax);

    alpha_f=atan2(vf(2),max(abs(vf(1)),0.1));
    alpha_r=atan2(vr(2),max(abs(vr(1)),0.1));

    ax_est=Fx_vehicle/m+vy*wz;

    Ffz=m*g*lr/L - m*ax_est*h/L;
    Frz=m*g*lf/L + m*ax_est*h/L;

    Fy_f=-Cf*alpha_f*Ffz;
    Fy_r=-Cr*alpha_r*Frz;

    dvx=(Fx_vehicle - Fy_f*sin(delta))/m;
    dvy=(Fy_f*cos(delta)+Fy_r)/m;
    dwz=(lf*Fy_f*cos(delta) - lr*Fy_r)/Jz;

    a_cog=[dvx;dvy;0];
    alpha_vec=[0;0;dwz];

    a_imu=a_cog + cross(omega,cross(omega,Rcog)) + cross(alpha_vec,Rcog);
    v_imu=v_cog + cross(omega,Rcog);

    omega_rl=vx/Rwheel;
    omega_rr=vx/Rwheel;

    Z(:,k)=[a_imu(1:2); v_imu(1:2); wz; omega_rl; omega_rr];
end

%% ===== z mean =====
z_pred=zeros(length(z),1);
for k=1:nSP
    w=(k==1)*W0 + (k>1)*Wi;
    z_pred=z_pred + w*Z(:,k);
end

%% ===== SENSOR SELECTION =====
valid_idx=true(length(z),1);

if ~isnan(z(IDX_VX))
    valid_idx(IDX_WRL)=false;
    valid_idx(IDX_WRR)=false;
else
    valid_idx(IDX_VX)=false;
end

valid_idx=valid_idx & ~isnan(z);

z_used=z(valid_idx);
z_pred_used=z_pred(valid_idx);
Z_used=Z(valid_idx,:);
R_used=R(valid_idx,valid_idx);

%% ===== S =====
S_cov=zeros(length(z_used));
for k=1:nSP
    w=(k==1)*W0 + (k>1)*Wi;
    dz=Z_used(:,k)-z_pred_used;
    S_cov=S_cov + w*(dz*dz');
end

S_cov=S_cov + R_used;
S_cov=(S_cov+S_cov')/2 + 1e-9*eye(size(S_cov));

%% ===== Pxz =====
Pxz=zeros(n,length(z_used));
for k=1:nSPx
    w=(k==1)*W0 + (k>1)*Wi;
    dx=SPx_new(:,k)-x_pred;
    dz=Z_used(:,k)-z_pred_used;
    Pxz=Pxz + w*(dx*dz');
end

%% ===== UPDATE =====
K=Pxz/S_cov;

x=x_pred + K*(z_used - z_pred_used);
Pk=P_pred - K*S_cov*K';
Pk=(Pk+Pk')/2 + 1e-9*eye(n);

%% ===== OUTPUT =====
xhat=x;
P=Pk;
dxdt=dxdt_model;

innovation=zeros(length(z),1);
innovation(valid_idx)=z_used - z_pred_used;

K_out=zeros(n,length(z));
K_out(:,valid_idx)=K;

S_out=zeros(length(z));
S_out(valid_idx,valid_idx)=S_cov;

z_pred_out=z_pred;

end

== matlab function generic_Truck_And_Trailer/TruckMaker/Subsystem1/ONE_TRACK_MODEL_TRACTOR_UKF/MATLAB Function1 ==
  data: z input; u input; xhat output; Q input; R input; Ts input; data input; P output; dxdt output; innovation output; K_out output; S_out output; z_pred_out output
function [xhat, P, dxdt, innovation, K_out, S_out, z_pred_out] = UKF_OneTrack_IMU(z, u, Q, R, Ts,data)

persistent x Pk dxdt_old t p_nom Pp

if isempty(x)
    x = [15;0.1;0.1;7.5;7.5];
end
if isempty(Pk)
    Pk = diag([0.1 0.1 0.1 5 5]);
end
if isempty(dxdt_old)
    dxdt_old = zeros(5,1);
end
if isempty(t)
    t = 0;
end
if isempty(p_nom)
    p_nom = [6800; 12994.917];
    Pp = diag([5000, 20000]).^2;
end

T_sim = 0.001;
t = t + T_sim;
t=data;

if t < 30
    xhat = x;
    P = Pk;
    dxdt = dxdt_old;
    innovation = zeros(length(z),1);
    K_out = zeros(length(x), length(z));
    S_out = eye(length(z));
    z_pred_out = zeros(length(z),1);
    return
end

IDX_VX  = 3; 
IDX_WRL = 6; 
IDX_WRR = 7;

g  = 9.82;

p_cog = [3.473;0;0.925];
p_fax = [4.520;0;0.490];
p_rax = [0.950;0;0.490];
p_imu = [3.600;0;1.000];

lf = abs(p_fax(1)-p_cog(1));
lr = abs(p_cog(1)-p_rax(1));
L  = lf + lr;
h  = p_cog(3);

Rfax = p_fax - p_cog; Rfax(3) = -p_cog(3);
Rrax = p_rax - p_cog; Rrax(3) = -p_cog(3);
Rcog = p_imu - p_cog;

delta = u(1);
T_rl  = u(2);
T_rr  = u(3);
Rwheel = 0.505;
Fx_vehicle = (T_rl + T_rr)/Rwheel;

n  = length(x);
np = length(p_nom);
nSPx = 2*n + 1;
nSPp = 2*np;
nSP  = nSPx + nSPp;

W0 = 1 - (n + np)/3;
Wi = (1 - W0)/(2*(n + np));
gamma = sqrt((n + np)/(1 - W0));

%% ===== STATE SIGMA =====
Pk = (Pk + Pk')/2 + 1e-9*eye(n);
Sx = chol(Pk,'lower');

X = zeros(n,nSPx);
X(:,1) = x;
for i=1:n
    X(:,i+1)   = x + gamma*Sx(:,i);
    X(:,i+1+n) = x - gamma*Sx(:,i);
end

%% ===== PARAM SIGMA =====
Pp = (Pp + Pp')/2 + 1e-9*eye(np);
Sp = chol(Pp,'lower');

SPp = zeros(np,nSPp);
for i=1:np
    SPp(:,i)    = p_nom + gamma*Sp(:,i);
    SPp(:,i+np) = p_nom - gamma*Sp(:,i);
end

%% ===== PREDICTION =====
X_prop = zeros(n,nSP);
dxdt_model = zeros(5,1);

for k=1:nSP
    if k <= nSPx
        Xk = X(:,k); 
        pk = p_nom;
    else
        Xk = x; 
        pk = SPp(:,k-nSPx);
    end

    vx=Xk(1); vy=Xk(2); wz=Xk(3); Cf=Xk(4); Cr=Xk(5);
    m=pk(1); Jz=pk(2);

    v_cog=[vx;vy;0]; 
    omega=[0;0;wz];

    Rotf=[cos(delta) -sin(delta) 0;
          sin(delta)  cos(delta)  0; 
           0          0          1];

    vf=Rotf.'*(v_cog+cross(omega,Rfax));
    vr=v_cog+cross(omega,Rrax);

    alpha_f=atan2(vf(2),max(abs(vf(1)),0.1));
    alpha_r=atan2(vr(2),max(abs(vr(1)),0.1));

    ax_est=Fx_vehicle/m+vy*wz;

    Ffz=m*g*lr/L - m*ax_est*h/L;
    Frz=m*g*lf/L + m*ax_est*h/L;

    Fy_f=-Cf*alpha_f*Ffz;
    Fy_r=-Cr*alpha_r*Frz;

    dvx=(Fx_vehicle - Fy_f*sin(delta))/m + vy*wz;
    dvy=(Fy_f*cos(delta)+Fy_r)/m - vx*wz;
    dwz=(lf*Fy_f*cos(delta) - lr*Fy_r)/Jz;

    if k==1
        dxdt_model=[dvx;dvy;dwz;0;0];
    end

    X_prop(:,k)=[vx+Ts*dvx; vy+Ts*dvy; wz+Ts*dwz; Cf; Cr];
end

%% ===== MEAN =====
x_pred=zeros(n,1);
for k=1:nSP
    w=(k==1)*W0 + (k>1)*Wi;
    x_pred=x_pred + w*X_prop(:,k);
end

%% ===== COV =====
P_pred=zeros(n);
for k=1:nSPx
    w=(k==1)*W0 + (k>1)*Wi;
    dx=X_prop(:,k)-x_pred;
    P_pred=P_pred + w*(dx*dx');
end
P_pred=P_pred + Q*Ts;

%% ===== NEW SIGMA POINTS =====
P_pred=(P_pred+P_pred')/2 + 1e-9*eye(n);
Sx=chol(P_pred,'lower');

SPx_new=zeros(n,nSPx);
SPx_new(:,1)=x_pred;

for i=1:n
    SPx_new(:,i+1)  =x_pred+gamma*Sx(:,i);
    SPx_new(:,i+1+n) =x_pred-gamma*Sx(:,i);
end

%% ===== MEASUREMENT =====
Z=zeros(length(z),nSP);

for k=1:nSP
    if k<=nSPx
        Xk=SPx_new(:,k);
        pk=p_nom;
    else
        Xk=x_pred;
        pk=SPp(:,k-nSPx);
    end

    vx=Xk(1); vy=Xk(2); wz=Xk(3);
    Cf=Xk(4); Cr=Xk(5);

    m=pk(1); Jz=pk(2);

    v_cog=[vx;vy;0]; omega=[0;0;wz];
    Rotf=[cos(delta) -sin(delta) 0; sin(delta) cos(delta) 0; 0 0 1];

    vf=Rotf.'*(v_cog+cross(omega,Rfax));
    vr=v_cog+cross(omega,Rrax);

    alpha_f=atan2(vf(2),max(abs(vf(1)),0.1));
    alpha_r=atan2(vr(2),max(abs(vr(1)),0.1));

    ax_est=Fx_vehicle/m+vy*wz;

    Ffz=m*g*lr/L - m*ax_est*h/L;
    Frz=m*g*lf/L + m*ax_est*h/L;

    Fy_f=-Cf*alpha_f*Ffz;
    Fy_r=-Cr*alpha_r*Frz;

    dvx=(Fx_vehicle - Fy_f*sin(delta))/m;
    dvy=(Fy_f*cos(delta)+Fy_r)/m;
    dwz=(lf*Fy_f*cos(delta) - lr*Fy_r)/Jz;

    a_cog=[dvx;dvy;0];
    alpha_vec=[0;0;dwz];

    a_imu=a_cog + cross(omega,cross(omega,Rcog)) + cross(alpha_vec,Rcog);
    v_imu=v_cog + cross(omega,Rcog);

    omega_rl=vx/Rwheel;
    omega_rr=vx/Rwheel;

    Z(:,k)=[a_imu(1:2); v_imu(1:2); wz; omega_rl; omega_rr];
end

%% ===== z mean =====
z_pred=zeros(length(z),1);
for k=1:nSP
    w=(k==1)*W0 + (k>1)*Wi;
    z_pred=z_pred + w*Z(:,k);
end

%% ===== SENSOR SELECTION =====
valid_idx=true(length(z),1);

if ~isnan(z(IDX_VX))
    valid_idx(IDX_WRL)=false;
    valid_idx(IDX_WRR)=false;
else
    valid_idx(IDX_VX)=false;
end

valid_idx=valid_idx & ~isnan(z);

z_used=z(valid_idx);
z_pred_used=z_pred(valid_idx);
Z_used=Z(valid_idx,:);
R_used=R(valid_idx,valid_idx);

%% ===== S =====
S_cov=zeros(length(z_used));
for k=1:nSP
    w=(k==1)*W0 + (k>1)*Wi;
    dz=Z_used(:,k)-z_pred_used;
    S_cov=S_cov + w*(dz*dz');
end

S_cov=S_cov + R_used;
S_cov=(S_cov+S_cov')/2 + 1e-9*eye(size(S_cov));

%% ===== Pxz =====
Pxz=zeros(n,length(z_used));
for k=1:nSPx
    w=(k==1)*W0 + (k>1)*Wi;
    dx=SPx_new(:,k)-x_pred;
    dz=Z_used(:,k)-z_pred_used;
    Pxz=Pxz + w*(dx*dz');
end

%% ===== UPDATE =====
K=Pxz/S_cov;

x=x_pred + K*(z_used - z_pred_used);
Pk=P_pred - K*S_cov*K';
Pk=(Pk+Pk')/2 + 1e-9*eye(n);

%% ===== OUTPUT =====
xhat=x;
P=Pk;
dxdt=dxdt_model;

innovation=zeros(length(z),1);
innovation(valid_idx)=z_used - z_pred_used;

K_out=zeros(n,length(z));
K_out(:,valid_idx)=K;

S_out=zeros(length(z));
S_out(valid_idx,valid_idx)=S_cov;

z_pred_out=z_pred;

end
